simulink model "BPSKImageTransferModificarCuantificador"  (R2016a)
settings: Solver=VariableStepDiscrete  SolverMode=SingleTasking  StartTime=0.0  StopTime=420800  RelTol=1e-3
libraries: commlibv2 x8, commutil2 x4, commcnvcod2 x4, commdigbbndpm3 x3, commchan3 x1, commhdledac x1, commhdllib x1, commsink2 x1, commdigbbnd2 x1, dspstat3 x1
settings Model: Creator=Glynis  LastModifiedBy=Glynis
settings DataIOCC: LimitDataPoints=on  SaveOutput=off  SaveTime=off
settings OptimizationCC: BooleanDataType=off  DefaultParameterBehavior=Inlined  LocalBlockOutputs=off
settings DebuggingCC: AlgebraicLoopMsg=error  SingleTaskRateTransMsg=error  AllowSymbolicDim=off
settings ConfigComp: CovModelRefEnable=Off  CovSFcnEnable=off

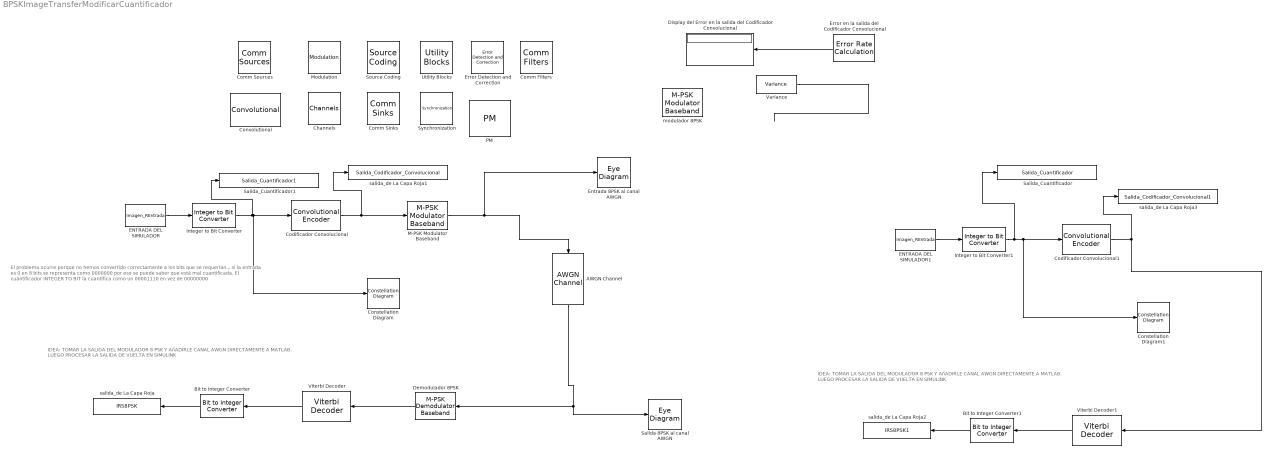
== system BPSKImageTransferModificarCuantificador ==
  note: El problema ocurre porque no hemos convertido correctamente a los bits que se requerían...
      | si la entrada es 0 en 8 bits se representa como 0000000 por eso se puede saber que
      | está mal cuantificada.
      |
      | El cuantificador INTEGER TO BIT la cuantifica como un
      | 00001110
      | en vez de
      | 00000000
  note: IDEA: TOMAR LA SALIDA DEL MODULADOR 8 PSK Y AñADIRLE CANAL AWGN DIRECTAMENTE A MATLAB. LUEGO PROCESAR LA SALIDA DE VUELTA EN SIMULINK
  note: IDEA: TOMAR LA SALIDA DEL MODULADOR 8 PSK Y AñADIRLE CANAL AWGN DIRECTAMENTE A MATLAB. LUEGO PROCESAR LA SALIDA DE VUELTA EN SIMULINK
  AWGN Channel : commchan3/AWGN Channel  InputProcessing=Columns as channels (frame based)  seed=654  noiseMode="Signal to noise ratio  (Eb/No)"  EbNodB=100  EsNodB=10  SNRdB=10  bitsPerSym=8  Ps=1000  Tsym=1  variance=1
  Bit to Integer Converter : commutil2/Bit to Integer Converter  nbits=8  bitOrder=MSB first  signedOutputValues=Unsigned  outDtype=Inherit via internal rule  outDtypeSigned=Inherit via internal rule
  Bit to Integer Converter1 : commutil2/Bit to Integer Converter  nbits=8  bitOrder=MSB first  signedOutputValues=Unsigned  outDtype=Inherit via internal rule  outDtypeSigned=Inherit via internal rule
  Channels : commlibv2/Channels
  Codificador Convolucional : commcnvcod2/Convolutional Encoder  trellis=poly2trellis(7, [171 133])  opMode=Truncated (reset every frame)  DelayedResetAction=on  hasIniStPort=off  hasFinStPort=off  usePuncVector=off  punctureVector=[1; 1; 0; 1; 0; 1]  reset=Unused parameter value
  Codificador Convolucional1 : commcnvcod2/Convolutional Encoder  trellis=poly2trellis(7, [171 133])  opMode=Truncated (reset every frame)  DelayedResetAction=on  hasIniStPort=off  hasFinStPort=off  usePuncVector=off  punctureVector=[1; 1; 0; 1; 0; 1]  reset=Unused parameter value
  Comm Filters : commlibv2/Comm Filters
  Comm Sinks : commlibv2/Comm Sinks
  Comm Sources : commlibv2/Comm Sources
  Constellation Diagram : ConstellationDiagram
  Constellation Diagram1 : ConstellationDiagram
  Convolutional : commhdledac/Convolutional
  Demodulador 8PSK : commdigbbndpm3/M-PSK Demodulator Baseband  M=8  OutType=Integer  DecType=Hard decision  VarSource=Dialog  Variance=1  Dec=Gray  Mapping=[0:7]  Ph=pi/8  outDtype1=Inherit via internal rule  outDtype2=Inherit via internal rule  derotateFactorWordLen=16  derotateFactorDataTypeStr=Inherit: Same word length as input  derotateFactorLastDataTypeStr=Inherit: Same word length as input
  Display del Error en la salida del Codificador Convolucional : Display
  ENTRADA DEL SIMULADOR : FromWorkspace  VariableName=Imagen_REntrada  SampleTime=1  OutputAfterFinalValue=Holding final value
  ENTRADA DEL SIMULADOR1 : FromWorkspace  VariableName=Imagen_REntrada  SampleTime=1  OutputAfterFinalValue=Holding final value
  Entrada 8PSK al canal AWGN : EyeDiagram
  Error Detection and Correction : commhdllib/Error Detection and Correction
  Error en la salida del Codificador Convolucional : commsink2/Error Rate Calculation  N=0  st_delay=0  cp_mode=Entire frame  subframe=[]  PMode=Port  WsName=ErrorVec  RsMode2=off  stop=off  numErr=100  maxBits=1e6
  Integer to Bit Converter : commutil2/Integer to Bit Converter  nbits=8  signedInputValues=Unsigned  bitOrder=MSB first  outDtype=Inherit via internal rule
  Integer to Bit Converter1 : commutil2/Integer to Bit Converter  nbits=8  signedInputValues=Unsigned  bitOrder=MSB first  outDtype=Inherit via internal rule
  M-PSK Modulator Baseband : commdigbbndpm3/M-PSK Modulator Baseband  M=8  InType=Integer  Enc=Gray  Mapping=[0:7]  Ph=pi/8  outDtype=double  outWordLen=16  outUDDataType=sfix(16)  outFracLenMode=Best precision  outFracLen=15  outDataTypeStr=double  outLastDataTypeStr=double
  Modulation : commlibv2/Modulation
  PM : commdigbbnd2/PM
  Salida 8PSK al canal AWGN : EyeDiagram
  Salida_Cuantificador : ToWorkspace  VariableName=Salida_Cuantificador  SampleTime=-1
      settings: Save2DSignal=2-D array (concatenate along first dimension)
  Salida_Cuantificador1 : ToWorkspace  VariableName=Salida_Cuantificador1  SampleTime=-1
      settings: Save2DSignal=2-D array (concatenate along first dimension)
  Source Coding : commlibv2/Source Coding
  Synchronization : commlibv2/Synchronization
  Utility Blocks : commlibv2/Utility Blocks
  Variance : dspstat3/Variance  run=off  reset_popup=None  InputProcessing=Columns as channels (frame based)  directionMode=Each column  dimension=1  roiEnable=off  roiType=Rectangles  roiPortion=Entire ROI  roiOutput=Individual statistics for each ROI  roiFlag=off  roundingMode=Floor  overflowMode=off
  Viterbi Decoder : commcnvcod2/Viterbi Decoder  trellis=poly2trellis(7, [171 133])  isPunctured=off  punctureVector=[1; 1; 0; 1; 0; 1]  erasures=off  dectype=Hard decision  nsdecb=4  runSigValErrCheck=off  tbdepth=34  opmode=Continuous  reset=off  delayedResetAction=on  smWordLength=16  outDataType=Smallest unsigned integer
  Viterbi Decoder1 : commcnvcod2/Viterbi Decoder  trellis=poly2trellis(7, [171 133])  isPunctured=off  punctureVector=[1; 1; 0; 1; 0; 1]  erasures=off  dectype=Hard decision  nsdecb=4  runSigValErrCheck=off  tbdepth=34  opmode=Continuous  reset=off  delayedResetAction=on  smWordLength=16  outDataType=Smallest unsigned integer
  modulador 8PSK : commdigbbndpm3/M-PSK Modulator Baseband  M=8  InType=Integer  Enc=Gray  Mapping=[0:7]  Ph=pi/8  outDtype=double  outWordLen=16  outUDDataType=sfix(16)  outFracLenMode=Best precision  outFracLen=15  outDataTypeStr=double  outLastDataTypeStr=double
  salida_de La Capa Roja : ToWorkspace  VariableName=IRS8PSK  SampleTime=-1
      settings: Save2DSignal=2-D array (concatenate along first dimension)
  salida_de La Capa Roja1 : ToWorkspace  VariableName=Salida_Codificador_Convolucional  SampleTime=-1
      settings: Save2DSignal=2-D array (concatenate along first dimension)
  salida_de La Capa Roja2 : ToWorkspace  VariableName=IRS8PSK1  SampleTime=-1
      settings: Save2DSignal=2-D array (concatenate along first dimension)
  salida_de La Capa Roja3 : ToWorkspace  VariableName=Salida_Codificador_Convolucional1  SampleTime=-1
      settings: Save2DSignal=2-D array (concatenate along first dimension)
  wires:
  Viterbi Decoder/1 -> Bit to Integer Converter/1
  Demodulador 8PSK/1 -> Viterbi Decoder/1
  Bit to Integer Converter/1 -> salida_de La Capa Roja/1
  ENTRADA DEL SIMULADOR/1 -> Integer to Bit Converter/1
  AWGN Channel/1 -> Salida 8PSK al canal AWGN/1, Demodulador 8PSK/1
  M-PSK Modulator Baseband/1 -> Entrada 8PSK al canal AWGN/1, AWGN Channel/1
  Codificador Convolucional/1 -> M-PSK Modulator Baseband/1, salida_de La Capa Roja1/1
  Error en la salida del Codificador Convolucional/1 -> Display del Error en la salida del Codificador Convolucional/1
  Variance/1 -> ?
  ? -> Variance/1
  Viterbi Decoder1/1 -> Bit to Integer Converter1/1
  Bit to Integer Converter1/1 -> salida_de La Capa Roja2/1
  ENTRADA DEL SIMULADOR1/1 -> Integer to Bit Converter1/1
  Codificador Convolucional1/1 -> Viterbi Decoder1/1, salida_de La Capa Roja3/1
  Integer to Bit Converter1/1 -> Salida_Cuantificador/1, Constellation Diagram1/1, Codificador Convolucional1/1
  Integer to Bit Converter/1 -> Salida_Cuantificador1/1, Constellation Diagram/1, Codificador Convolucional/1
